simulink library "RailCab"  (Simulink 7.4)
settings: Solver=ode45  StartTime=0.0  StopTime=10.0  RelTol=1e-3
libraries: Communication x1
settings Model: Creator=dread  LastModifiedBy=dread

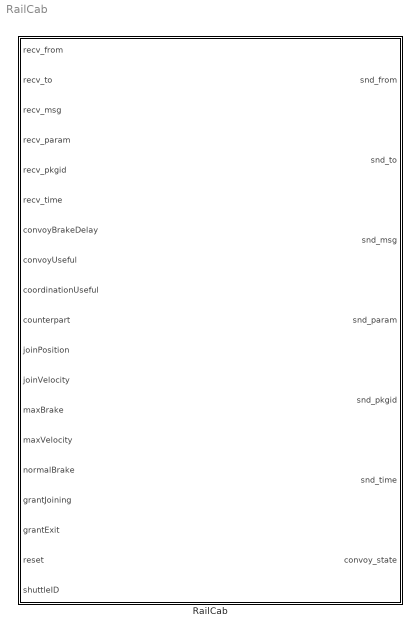
== system RailCab ==
  RailCab : Subsystem

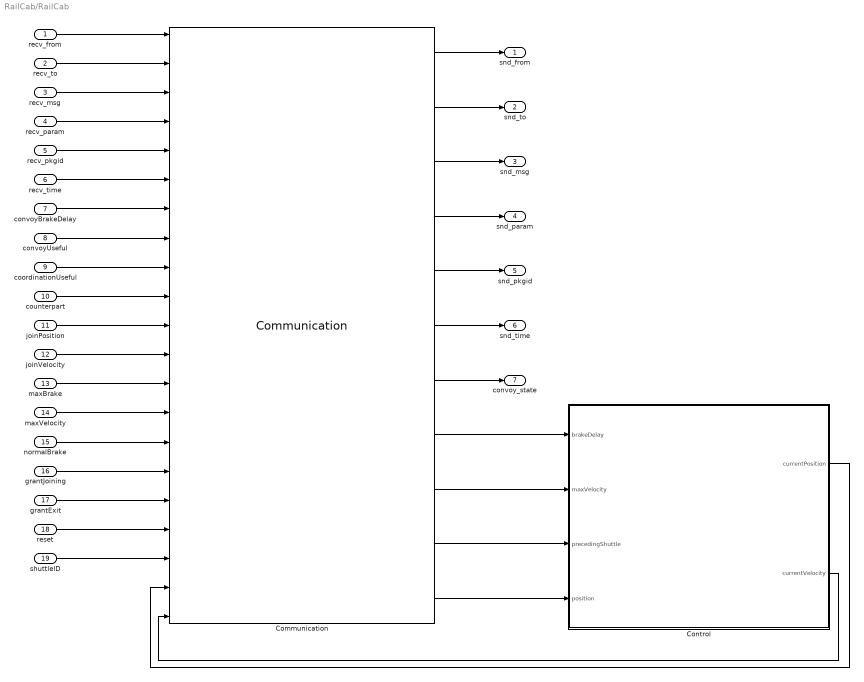
== system RailCab/RailCab ==
  recv_from : Inport  DataType=uint8  OutDataType=fixdt(1, 16)  OutScaling=2^0  OutDataTypeStr=uint8
  recv_to : Inport  Port=2  DataType=uint8  OutDataType=fixdt(1, 16)  OutScaling=2^0  OutDataTypeStr=uint8
  recv_msg : Inport  Port=3  DataType=uint16  OutDataType=fixdt(1, 16)  OutScaling=2^0  OutDataTypeStr=uint16
  recv_param : Inport  Port=4  DataType=double  OutDataType=fixdt(1, 16)  OutScaling=2^0  OutDataTypeStr=double
  recv_pkgid : Inport  Port=5  DataType=uint32  OutDataType=fixdt(1, 16)  OutScaling=2^0  OutDataTypeStr=uint32
  recv_time : Inport  Port=6  DataType=double  OutDataType=fixdt(1, 16)  OutScaling=2^0  OutDataTypeStr=double
  convoyBrakeDelay : Inport  Port=7  DataType=double  OutDataType=fixdt(1, 16)  OutScaling=2^0  OutDataTypeStr=double
  convoyUseful : Inport  Port=8  DataType=boolean  OutDataType=fixdt(1, 16)  OutScaling=2^0  OutDataTypeStr=boolean
  coordinationUseful : Inport  Port=9  DataType=boolean  OutDataType=fixdt(1, 16)  OutScaling=2^0  OutDataTypeStr=boolean
  counterpart : Inport  Port=10  DataType=double  OutDataType=fixdt(1, 16)  OutScaling=2^0  OutDataTypeStr=double
  joinPosition : Inport  Port=11  DataType=double  OutDataType=fixdt(1, 16)  OutScaling=2^0  OutDataTypeStr=double
  joinVelocity : Inport  Port=12  DataType=double  OutDataType=fixdt(1, 16)  OutScaling=2^0  OutDataTypeStr=double
  maxBrake : Inport  Port=13  DataType=double  OutDataType=fixdt(1, 16)  OutScaling=2^0  OutDataTypeStr=double
  maxVelocity : Inport  Port=14  DataType=double  OutDataType=fixdt(1, 16)  OutScaling=2^0  OutDataTypeStr=double
  normalBrake : Inport  Port=15  DataType=double  OutDataType=fixdt(1, 16)  OutScaling=2^0  OutDataTypeStr=double
  grantJoining : Inport  Port=16  OutDataType=fixdt(1, 16)  OutScaling=2^0
  grantExit : Inport  Port=17  OutDataType=fixdt(1, 16)  OutScaling=2^0
  reset : Inport  Port=18  DataType=boolean  OutDataType=fixdt(1, 16)  OutScaling=2^0  OutDataTypeStr=boolean
  shuttleID : Inport  Port=19  DataType=uint8  OutDataType=fixdt(1, 16)  OutScaling=2^0  OutDataTypeStr=uint8
  Communication : Communication/Communication  SystemSampleTime=-1
  Control : Subsystem
  snd_from : Outport  DataType=uint8  OutDataType=fixdt(1, 16)  OutScaling=2^0  OutDataTypeStr=uint8
  snd_to : Outport  Port=2  DataType=uint8  OutDataType=fixdt(1, 16)  OutScaling=2^0  OutDataTypeStr=uint8
  snd_msg : Outport  Port=3  DataType=uint16  OutDataType=fixdt(1, 16)  OutScaling=2^0  OutDataTypeStr=uint16
  snd_param : Outport  Port=4  DataType=double  OutDataType=fixdt(1, 16)  OutScaling=2^0  OutDataTypeStr=double
  snd_pkgid : Outport  Port=5  DataType=uint32  OutDataType=fixdt(1, 16)  OutScaling=2^0  OutDataTypeStr=uint32
  snd_time : Outport  Port=6  DataType=double  OutDataType=fixdt(1, 16)  OutScaling=2^0  OutDataTypeStr=double
  convoy_state : Outport  Port=7  OutDataType=fixdt(1, 16)  OutScaling=2^0
  wires:
  Communication/10 -> Control/3(precedingShuttle)
  Communication/9 -> Control/2(maxVelocity)
  Control/1(currentPosition) -> Communication/20
  Control/2(currentVelocity) -> Communication/21
  Communication/11 -> Control/4(position)
  Communication/8 -> Control/1(brakeDelay)
  Communication/7 -> convoy_state/1
  recv_from/1 -> Communication/1
  recv_to/1 -> Communication/2
  recv_msg/1 -> Communication/3
  recv_param/1 -> Communication/4
  recv_pkgid/1 -> Communication/5
  recv_time/1 -> Communication/6
  maxBrake/1 -> Communication/13
  convoyBrakeDelay/1 -> Communication/7
  convoyUseful/1 -> Communication/8
  coordinationUseful/1 -> Communication/9
  counterpart/1 -> Communication/10
  joinPosition/1 -> Communication/11
  joinVelocity/1 -> Communication/12
  maxVelocity/1 -> Communication/14
  normalBrake/1 -> Communication/15
  grantJoining/1 -> Communication/16
  grantExit/1 -> Communication/17
  reset/1 -> Communication/18
  shuttleID/1 -> Communication/19
  Communication/6 -> snd_time/1
  Communication/5 -> snd_pkgid/1
  Communication/4 -> snd_param/1
  Communication/3 -> snd_msg/1
  Communication/2 -> snd_to/1
  Communication/1 -> snd_from/1

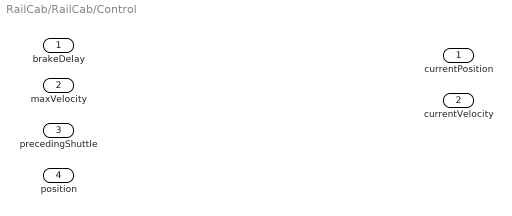
== system RailCab/RailCab/Control ==
  brakeDelay : Inport  OutDataType=fixdt(1, 16)  OutScaling=2^0
  maxVelocity : Inport  Port=2  OutDataType=fixdt(1, 16)  OutScaling=2^0
  precedingShuttle : Inport  Port=3  DataType=uint8  OutDataType=fixdt(1, 16)  OutScaling=2^0  OutDataTypeStr=uint8
  position : Inport  Port=4  PortDimensions=3  DataType=double  OutDataType=fixdt(1, 16)  OutScaling=2^0  OutDataTypeStr=double
  currentPosition : Outport  PortDimensions=2  DataType=double  OutDataType=fixdt(1, 16)  OutScaling=2^0  OutDataTypeStr=double
  currentVelocity : Outport  Port=2  DataType=double  OutDataType=fixdt(1, 16)  OutScaling=2^0  OutDataTypeStr=double
